simulink library "dclink_for_three_levels"  (R2025b)
settings: Solver=VariableStepAuto  StartTime=0.0  StopTime=10.0  RelTol=1e-3
libraries: fl_lib x27, nesl_utility x14, $bdroot x1
settings Model: Creator=dbagn  LastModifiedBy=dbagn

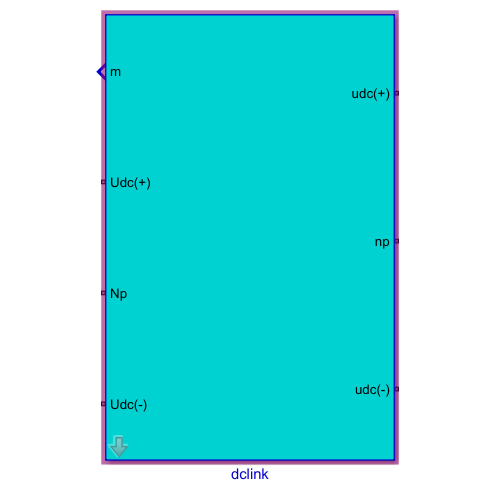
[thumbnail: Simulink's stored preview of the top-level diagram]
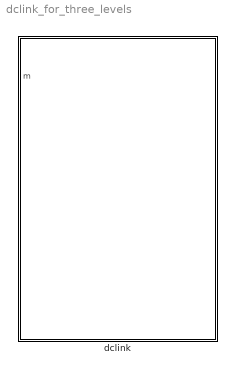
== system dclink_for_three_levels ==
  dclink : Subsystem  mask{Cdc1_m=7.2e-3, Cdc2_m=7.2e-3, Rudc_measure=107e3, Vdc_scale=1070, Vdc1_m_init=1070/2, Vdc2_m_init=1070/2}
      mask prompts: Cdc1_m "Cdc1 [F]"; Cdc2_m "Cdc2 [F]"; Vdc_scale "Vdc_scale [V]"; Vdc1_m_init "Vdc1 init [V]"; Vdc2_m_init "Vdc2 init [V]"

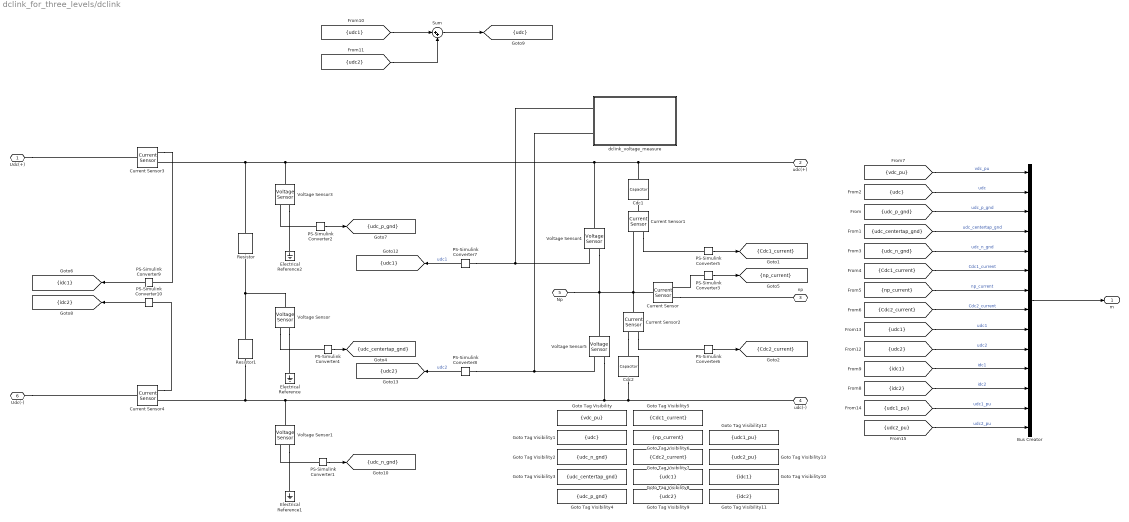
== system dclink_for_three_levels/dclink ==
  Bus Creator : BusCreator  Inputs=14
  Cdc1 : fl_lib/Electrical/Electrical Elements/Capacitor  c=Cdc1_m F  r=2e-3 Ohm  g=0 1/Ohm  i_specify=off  i_priority=High  i=0 A  i_nominal_specify=off  i_nominal_value=1  i_nominal_unit=A  v_specify=on  v_priority=High  v=Vdc1_m_init V  v_nominal_specify=off  v_nominal_value=1  v_nominal_unit=V  vc_specify=off  vc_priority=High  vc=0 V  vc_nominal_specify=off  vc_nominal_value=1  vc_nominal_unit=V
  Cdc2 : fl_lib/Electrical/Electrical Elements/Capacitor  c=Cdc2_m F  r=2e-3 Ohm  g=0 1/Ohm  i_specify=off  i_priority=High  i=0 A  i_nominal_specify=off  i_nominal_value=1  i_nominal_unit=A  v_specify=on  v_priority=High  v=Vdc2_m_init V  v_nominal_specify=off  v_nominal_value=1  v_nominal_unit=V  vc_specify=off  vc_priority=High  vc=0 V  vc_nominal_specify=off  vc_nominal_value=1  vc_nominal_unit=V
  Current Sensor{,1..4} (5 alike) : fl_lib/Electrical/Electrical Sensors/Current Sensor
  Electrical Reference : fl_lib/Electrical/Electrical Elements/Electrical Reference
  Electrical Reference1 : fl_lib/Electrical/Electrical Elements/Electrical Reference
  Electrical Reference2 : fl_lib/Electrical/Electrical Elements/Electrical Reference
  Goto Tag Visibility : GotoTagVisibility  GotoTag=vdc_pu
  Goto Tag Visibility1 : GotoTagVisibility  GotoTag=udc
  Goto Tag Visibility10 : GotoTagVisibility  GotoTag=idc1
  Goto Tag Visibility11 : GotoTagVisibility  GotoTag=idc2
  Goto Tag Visibility12 : GotoTagVisibility  GotoTag=udc1_pu
  Goto Tag Visibility13 : GotoTagVisibility  GotoTag=udc2_pu
  Goto Tag Visibility2 : GotoTagVisibility  GotoTag=udc_n_gnd
  Goto Tag Visibility3 : GotoTagVisibility  GotoTag=udc_centertap_gnd
  Goto Tag Visibility4 : GotoTagVisibility  GotoTag=udc_p_gnd
  Goto Tag Visibility5 : GotoTagVisibility  GotoTag=Cdc1_current
  Goto Tag Visibility6 : GotoTagVisibility  GotoTag=np_current
  Goto Tag Visibility7 : GotoTagVisibility  GotoTag=Cdc2_current
  Goto Tag Visibility8 : GotoTagVisibility  GotoTag=udc1
  Goto Tag Visibility9 : GotoTagVisibility  GotoTag=udc2
  PS-Simulink Converter{1..2,4,7..8} (5 alike) : nesl_utility/PS-Simulink Converter  PhysicalDomain=network_engine_domain  SubClassName=ps_output  LeftPortType=input  RightPortType=output  PseudoPeriodic=off  Frequencies=[]  VectorFormat=1-D array  Unit=V  AffineConversion=on
  PS-Simulink Converter{3,5..6,9..10} (5 alike) : nesl_utility/PS-Simulink Converter  PhysicalDomain=network_engine_domain  SubClassName=ps_output  LeftPortType=input  RightPortType=output  PseudoPeriodic=off  Frequencies=[]  VectorFormat=1-D array  Unit=A  AffineConversion=on
  Resistor : fl_lib/Electrical/Electrical Elements/Resistor  R=1e6 Ohm  i_specify=off  i_priority=None  i=0 A  i_nominal_specify=off  i_nominal_value=1  i_nominal_unit=A  v_specify=off  v_priority=None  v=0 V  v_nominal_specify=off  v_nominal_value=1  v_nominal_unit=V
  Resistor1 : fl_lib/Electrical/Electrical Elements/Resistor  R=1e6 Ohm  i_specify=off  i_priority=None  i=0 A  i_nominal_specify=off  i_nominal_value=1  i_nominal_unit=A  v_specify=off  v_priority=None  v=0 V  v_nominal_specify=off  v_nominal_value=1  v_nominal_unit=V
  Sum : Sum  Inputs=|++
  Voltage Sensor{,1,3..5} (5 alike) : fl_lib/Electrical/Electrical Sensors/Voltage Sensor
  dclink_voltage_measure : Subsystem
  Udc(+) : PMIOPort  Side=Right
  udc(+) : PMIOPort  Port=2  Side=Left
  np : PMIOPort  Port=3  Side=Left
  udc(-) : PMIOPort  Port=4  Side=Left
  Np : PMIOPort  Port=5  Side=Right
  Udc(-) : PMIOPort  Port=6  Side=Right
  m : Outport
  tag scope: Cdc1_current=scoped, Cdc2_current=scoped, idc1=scoped, idc2=scoped, np_current=scoped, udc1=scoped, udc2=scoped, udc=scoped, udc_centertap_gnd=scoped, udc_n_gnd=scoped, udc_p_gnd=scoped
  wires:
  PS-Simulink Converter2/1 -> [udc_p_gnd]
  PS-Simulink Converter1/1 -> [udc_n_gnd]
  PS-Simulink Converter5/1 -> [Cdc1_current]
  PS-Simulink Converter6/1 -> [Cdc2_current]
  PS-Simulink Converter4/1 -> [udc_centertap_gnd]
  PS-Simulink Converter3/1 -> [np_current]
  [vdc_pu] -> Bus Creator/1  "vdc_pu"
  [udc] -> Bus Creator/2  "udc"
  [udc_p_gnd] -> Bus Creator/3  "udc_p_gnd"
  [udc_centertap_gnd] -> Bus Creator/4  "udc_centertap_gnd"
  [udc_n_gnd] -> Bus Creator/5  "udc_n_gnd"
  [Cdc1_current] -> Bus Creator/6  "Cdc1_current"
  [np_current] -> Bus Creator/7  "np_current"
  [Cdc2_current] -> Bus Creator/8  "Cdc2_current"
  Bus Creator/1 -> m/1
  [udc1] -> Bus Creator/9  "udc1"
  PS-Simulink Converter8/1 -> [udc2]  "udc2"
  [udc2] -> Bus Creator/10  "udc2"
  PS-Simulink Converter7/1 -> [udc1]  "udc1"
  PS-Simulink Converter9/1 -> [idc1]
  PS-Simulink Converter10/1 -> [idc2]
  [idc1] -> Bus Creator/11  "idc1"
  [idc2] -> Bus Creator/12  "idc2"
  [udc1] -> Sum/1
  Sum/1 -> [udc]
  [udc2] -> Sum/2
  [udc1_pu] -> Bus Creator/13  "udc1_pu"
  [udc2_pu] -> Bus Creator/14  "udc2_pu"
  connections:
  Voltage Sensor/RConn2 -- Electrical Reference/LConn1
  Voltage Sensor3/RConn2 -- Electrical Reference2/LConn1
  Current Sensor4/RConn2 -- Resistor1/RConn1 -- Voltage Sensor1/LConn1 -- Voltage Sensor5/RConn2 -- Cdc2/RConn1 -- udc(-)/RConn1
  Voltage Sensor/RConn1 -- PS-Simulink Converter4/LConn1
  PS-Simulink Converter2/LConn1 -- Voltage Sensor3/RConn1
  Voltage Sensor1/RConn2 -- Electrical Reference1/LConn1
  Cdc1/LConn1 -- Voltage Sensor4/LConn1 -- Voltage Sensor3/LConn1 -- Current Sensor3/RConn2 -- Resistor/LConn1 -- udc(+)/RConn1
  Resistor1/LConn1 -- Voltage Sensor/LConn1 -- Resistor/RConn1
  PS-Simulink Converter1/LConn1 -- Voltage Sensor1/RConn1
  Current Sensor/RConn2 -- np/RConn1
  Current Sensor1/LConn1 -- Cdc1/RConn1
  Current Sensor2/RConn2 -- Cdc2/LConn1
  Current Sensor2/LConn1 -- Voltage Sensor5/LConn1 -- Voltage Sensor4/RConn2 -- Np/RConn1 -- Current Sensor1/RConn2 -- Current Sensor/LConn1
  Current Sensor1/RConn1 -- PS-Simulink Converter5/LConn1
  Current Sensor2/RConn1 -- PS-Simulink Converter6/LConn1
  PS-Simulink Converter3/LConn1 -- Current Sensor/RConn1
  PS-Simulink Converter7/LConn1 -- Voltage Sensor4/RConn1 -- dclink_voltage_measure/LConn1
  PS-Simulink Converter8/LConn1 -- dclink_voltage_measure/LConn2 -- Voltage Sensor5/RConn1
  Udc(-)/RConn1 -- Current Sensor4/LConn1
  Udc(+)/RConn1 -- Current Sensor3/LConn1
  Current Sensor3/RConn1 -- PS-Simulink Converter9/LConn1
  Current Sensor4/RConn1 -- PS-Simulink Converter10/LConn1

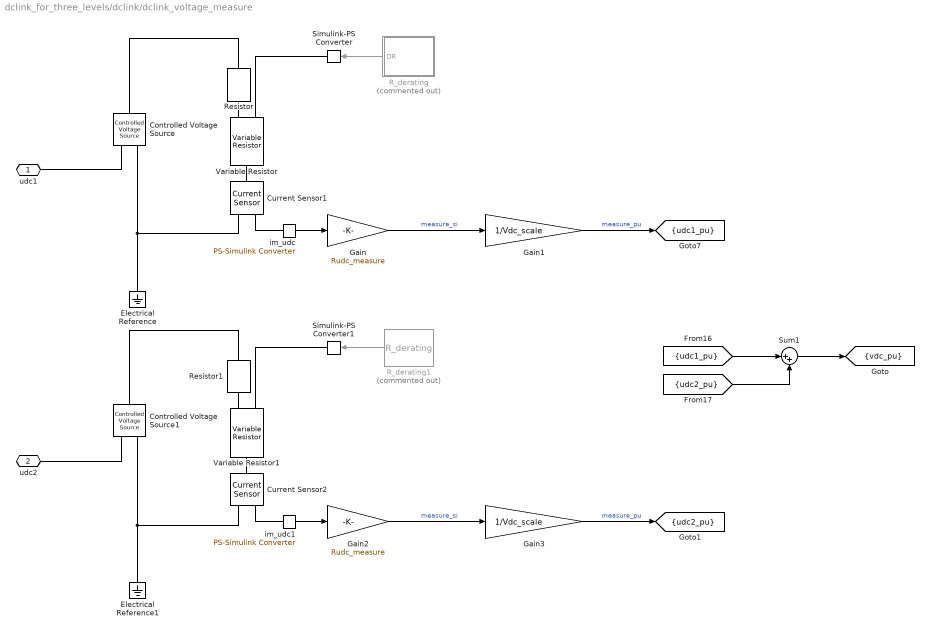
== system dclink_for_three_levels/dclink/dclink_voltage_measure ==
  Controlled Voltage Source : fl_lib/Electrical/Electrical Sources/Controlled Voltage Source
  Controlled Voltage Source1 : fl_lib/Electrical/Electrical Sources/Controlled Voltage Source
  Current Sensor1 : fl_lib/Electrical/Electrical Sensors/Current Sensor
  Current Sensor2 : fl_lib/Electrical/Electrical Sensors/Current Sensor
  Electrical Reference : fl_lib/Electrical/Electrical Elements/Electrical Reference
  Electrical Reference1 : fl_lib/Electrical/Electrical Elements/Electrical Reference
  Gain : Gain  Gain=Rudc_measure
  Gain1 : Gain  Gain=1/Vdc_scale
  Gain2 : Gain  Gain=Rudc_measure
  Gain3 : Gain  Gain=1/Vdc_scale
  R_derating : Subsystem  Commented=on
  R_derating1 : $bdroot/dclink/dclink_voltage_measure/R_derating  Commented=on  SystemSampleTime=-1  VariantActivationTime=update diagram  EmptyChoice=off  PassThrough=off  PassThroughVariantControl=(default)  EmptyChoiceVariantControl=(default)  AllowFlexibleInterface=on  Latency=0  AutoFrameSizeCalculation=off
  Resistor : fl_lib/Electrical/Electrical Elements/Resistor  R=Rudc_measure Ohm  i_specify=off  i_priority=None  i=0 A  i_nominal_specify=off  i_nominal_value=1  i_nominal_unit=A  v_specify=off  v_priority=None  v=0 V  v_nominal_specify=off  v_nominal_value=1  v_nominal_unit=V
  Resistor1 : fl_lib/Electrical/Electrical Elements/Resistor  R=Rudc_measure Ohm  i_specify=off  i_priority=None  i=0 A  i_nominal_specify=off  i_nominal_value=1  i_nominal_unit=A  v_specify=off  v_priority=None  v=0 V  v_nominal_specify=off  v_nominal_value=1  v_nominal_unit=V
  Simulink-PS Converter : nesl_utility/Simulink-PS Converter  PhysicalDomain=network_engine_domain  SubClassName=ps_input  LeftPortType=input  RightPortType=output  PseudoPeriodic=off  Frequencies=[]  NoiseDistribution=none  NoiseParameters=[]  Unit=Ohm  AffineConversion=off  FilteringAndDerivatives=provide  SimscapeFilterOrder=1  InputFilterTimeConstant=0.001  UdotUserProvided=0
  Simulink-PS Converter1 : nesl_utility/Simulink-PS Converter  PhysicalDomain=network_engine_domain  SubClassName=ps_input  LeftPortType=input  RightPortType=output  PseudoPeriodic=off  Frequencies=[]  NoiseDistribution=none  NoiseParameters=[]  Unit=Ohm  AffineConversion=off  FilteringAndDerivatives=provide  SimscapeFilterOrder=1  InputFilterTimeConstant=0.001  UdotUserProvided=0
  Sum1 : Sum  Inputs=|++
  Variable Resistor : fl_lib/Electrical/Electrical Elements/Variable Resistor  Rmin=0 Ohm  thermalEnable=false  thermal_mass=1 J/K  i_specify=off  i_priority=None  i=0 A  i_nominal_specify=off  i_nominal_value=1  i_nominal_unit=A  v_specify=off  v_priority=None  v=0 V  v_nominal_specify=off  v_nominal_value=1  v_nominal_unit=V  T_specify=off  T_priority=None  T=300 K  T_nominal_specify=off  T_nominal_value=1  T_nominal_unit=K
  Variable Resistor1 : fl_lib/Electrical/Electrical Elements/Variable Resistor  Rmin=0 Ohm  thermalEnable=false  thermal_mass=1 J/K  i_specify=off  i_priority=None  i=0 A  i_nominal_specify=off  i_nominal_value=1  i_nominal_unit=A  v_specify=off  v_priority=None  v=0 V  v_nominal_specify=off  v_nominal_value=1  v_nominal_unit=V  T_specify=off  T_priority=None  T=300 K  T_nominal_specify=off  T_nominal_value=1  T_nominal_unit=K
  im_udc : nesl_utility/PS-Simulink Converter  PhysicalDomain=network_engine_domain  SubClassName=ps_output  LeftPortType=input  RightPortType=output  PseudoPeriodic=off  Frequencies=[]  VectorFormat=1-D array  Unit=A  AffineConversion=on
  im_udc1 : nesl_utility/PS-Simulink Converter  PhysicalDomain=network_engine_domain  SubClassName=ps_output  LeftPortType=input  RightPortType=output  PseudoPeriodic=off  Frequencies=[]  VectorFormat=1-D array  Unit=A  AffineConversion=on
  udc1 : PMIOPort  Side=Left
  udc2 : PMIOPort  Port=2  Side=Left
  tag scope: udc1_pu=scoped, udc2_pu=scoped, vdc_pu=scoped
  wires:
  Gain/1 -> Gain1/1  "measure_si"
  im_udc/1 -> Gain/1
  Gain1/1 -> [udc1_pu]  "measure_pu"
  R_derating/1(DR) -> Simulink-PS Converter/1
  R_derating1/1 -> Simulink-PS Converter1/1
  Gain3/1 -> [udc2_pu]  "measure_pu"
  im_udc1/1 -> Gain2/1
  Gain2/1 -> Gain3/1  "measure_si"
  [udc1_pu] -> Sum1/1
  [udc2_pu] -> Sum1/2
  Sum1/1 -> [vdc_pu]
  connections:
  udc1/RConn1 -- Controlled Voltage Source/RConn1
  Resistor/RConn1 -- Variable Resistor/LConn2
  Current Sensor1/RConn1 -- im_udc/LConn1
  Current Sensor1/RConn2 -- Electrical Reference/LConn1 -- Controlled Voltage Source/RConn2
  Current Sensor1/LConn1 -- Variable Resistor/RConn1
  Simulink-PS Converter/RConn1 -- Variable Resistor/LConn1
  Controlled Voltage Source/LConn1 -- Resistor/LConn1
  Current Sensor2/RConn2 -- Controlled Voltage Source1/RConn2 -- Electrical Reference1/LConn1
  Controlled Voltage Source1/LConn1 -- Resistor1/LConn1
  Simulink-PS Converter1/RConn1 -- Variable Resistor1/LConn1
  Current Sensor2/RConn1 -- im_udc1/LConn1
  Resistor1/RConn1 -- Variable Resistor1/LConn2
  udc2/RConn1 -- Controlled Voltage Source1/RConn1
  Current Sensor2/LConn1 -- Variable Resistor1/RConn1

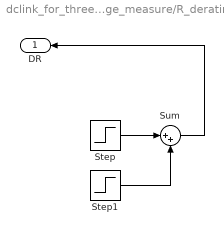
== system dclink_for_three_levels/dclink/dclink_voltage_measure/R_derating ==
  Step : Step  After=107.4e3/2  SampleTime=0
  Step1 : Step  Time=1.1  After=-107.4e3/2  SampleTime=0
  Sum : Sum  Inputs=|++
  DR : Outport
  wires:
  Step1/1 -> Sum/2
  Step/1 -> Sum/1
  Sum/1 -> DR/1
